simulink model "PID_LOOP_2024a"  (R2024a)
settings: Solver=FixedStepAuto  StartTime=0.0  StopTime=100  FixedStep=dt  RelTol=1e-3
model workspace (MAT data in the model file):
  Drag_Constants = 1
  mass = [5.51 5.51 5.51 1 1 1]
  mass_6a = [5 5 5 1 1 1]
values from neighbouring files (symbols this model uses):
  drag_wrench = [ ... (first row only)    [constants.m]    (also in constants.mat = [0.41 0 0 0 0 0 0 0.5 0 0 0 0 ... (36 elements, 6x6)])
  g = 9.8067    [constants.m]    (also in constants.mat = 9.80665)
  m = mc + mp    (= 6)    [calculate_inertia.m]    (also in constants.mat = 5.51; mass_properties.mat = 10)
  states_desired = [x_des;E_des]    [init.m]
  volume = 0.0074    [constants.m]    (also in constants.mat = 0.0073741788)
  volume_center = [0, 0, -0.07]    [constants.m]    (also in constants.mat = [0 0 0.1])
  water_density = 997    [constants.m]    (also in constants.mat = 1000)
  wrench = eval(w)    [calculate_wrench.m]    (also in constants.m = geometry_properties.wrench; constants.mat = [0 0 0 0 -0.7071 -0.7071 -0.7071 -0.7071 0 0 0 0 ... (48 ele; geometry_properties.mat = [0 0 -1 0.22 0.25 0 0 0 -1 -0.22 0.25 0 ... (48 elements, 6x; wrench.m)
undefined symbols (not defined in the file or in its folder): E0_est, kd, ki, kp, P, pwm_stop, v0_e_est, x0_e_est
libraries: slpidlib x7, simulink x3, shared6dof x1, sharedTrackingLibrary x1
settings Model: Creator=zenyn  LastModifiedBy=kjhaydon
settings DataIOCC: LoggingToFile=on
settings DebuggingCC: UnderSpecifiedDimensionMsg=warning

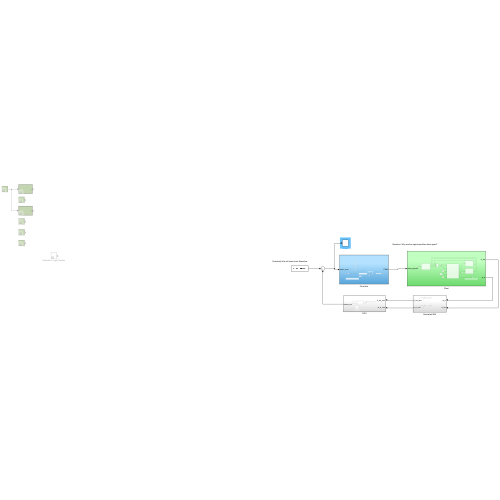
[thumbnail: Simulink's stored preview of the top-level diagram]
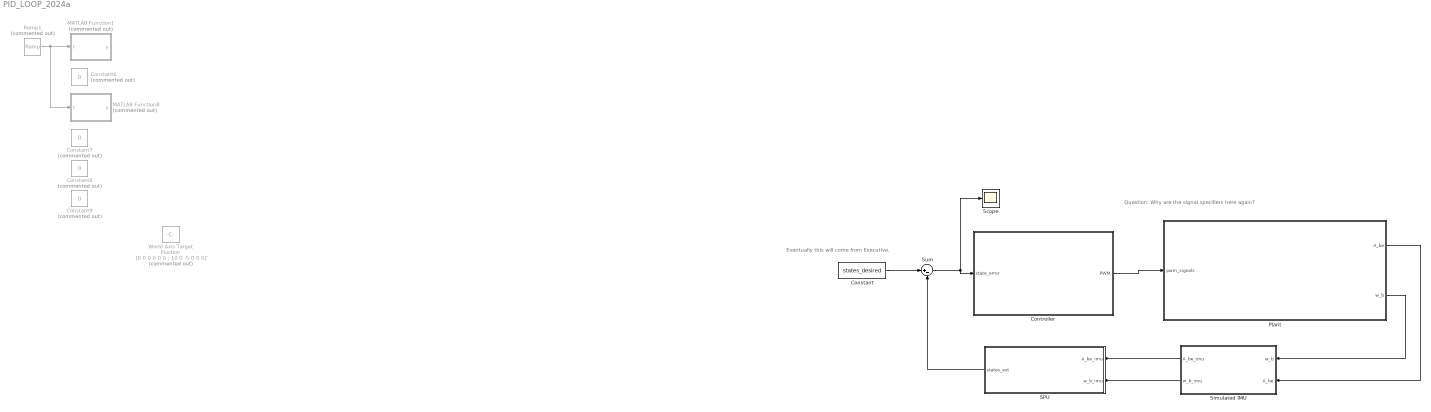
== system PID_LOOP_2024a ==
  note: Eventually this will come from Executive.
  note: Question: Why are the signal specifiers here again?
  Constant : Constant  Value=states_desired
  Constant{6..9} (4 alike) : Constant  Commented=on  Value=0
  Controller : Subsystem
  MATLAB Function1 : MATLAB Function  Commented=on  TreatAsAtomicUnit=on
  MATLAB Function8 : MATLAB Function  Commented=on  TreatAsAtomicUnit=on
  Plant : Subsystem
  Ramp1 : simulink/Sources/Ramp  Commented=on  slope=1  start=0  InitialOutput=0
  SPU : Subsystem
  Scope : Scope
  Simulated IMU : Subsystem
  Sum : Sum  Inputs=|+-
  World Axis Target Position : Constant  Commented=on  Value=[0 0 0 0 0 0 ; 10 0 -5 0 0 0]'
  wires:
  Sum/1 -> Scope/1, Controller/1(state_error)
  Ramp1/1 -> MATLAB Function8/1(t), MATLAB Function1/1(t)
  Simulated IMU/1(A_be_imu) -> SPU/1(A_be_imu)
  SPU/1(states_est) -> Sum/2
  Plant/2(w_b) -> Simulated IMU/1(w_b)
  Plant/1(A_be) -> Simulated IMU/2(A_be)
  Simulated IMU/2(w_b_imu) -> SPU/2(w_b_imu)
  Constant/1 -> Sum/1
  Controller/1(PWM) -> Plant/1(pwm_signals)

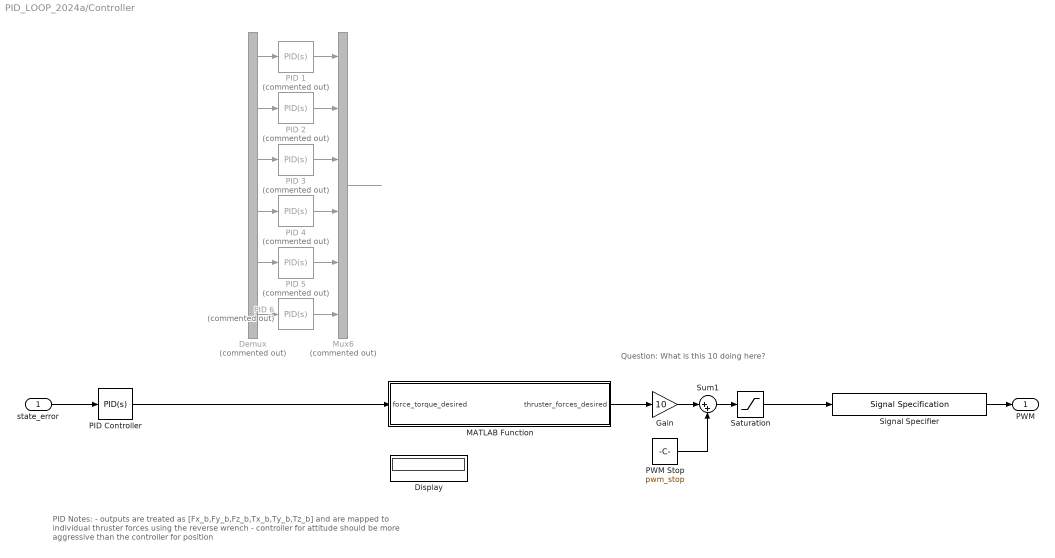
== system PID_LOOP_2024a/Controller ==
  note: Question: What is this 10 doing here?
  note: PID Notes:
      | - outputs are treated as [Fx_b,Fy_b,Fz_b,Tx_b,Ty_b,Tz_b] and are mapped to individual thruster forces using the reverse wrench
      | - controller for attitude should be more aggressive than the controller for position
  state_error : Inport
  Demux : Demux  Commented=on  Outputs=6
  Display : Display
  Gain : Gain  Gain=10
  MATLAB Function : MATLAB Function  TreatAsAtomicUnit=on
  Mux6 : Mux  Commented=on  Inputs=6
  PID 1 : slpidlib/PID Controller  Commented=on  Controller=PID  Form=Parallel  TimeDomain=Continuous-time  UseExternalTs=off  SampleTime=-1  IntegratorMethod=Forward Euler  FilterMethod=Forward Euler  ControllerParametersSource=internal  P=50  I=1  UseKiTs=off  D=80  UseExternalDerivativeSource=off  N=100  UseFilter=on  TunerSelectOption=Transfer Function Based (PID Tuner App)  InitialConditionSource=internal  InitialConditionForIntegrator=0  InitialConditionForFilter=0  DifferentiatorICPrevScaledInput=0  ExternalReset=none  TrackingMode=off  Kt=1  LimitOutput=off  SatLimitsSource=internal  UpperSaturationLimit=inf  LowerSaturationLimit=-inf  LinearizeAsGain=on  AntiWindupMode=none  Kb=1  LimitIntegrator=off  UpperIntegratorSaturationLimit=inf  LowerIntegratorSaturationLimit=-inf  POutMin=[]  POutMax=[]  IOutMin=[]  IOutMax=[]  DOutMin=[]  DOutMax=[]  NOutMin=[]  NOutMax=[]  SumOutMin=[]  SumOutMax=[]  SaturationOutMin=[]  SaturationOutMax=[]  PParamMin=[]  PParamMax=[]  IParamMin=[]  IParamMax=[]  DParamMin=[]  DParamMax=[]  NParamMin=[]  NParamMax=[]  KbParamMin=[]  KbParamMax=[]  KtParamMin=[]  KtParamMax=[]  KbOutMin=[]  KbOutMax=[]  KtOutMin=[]  KtOutMax=[]  IntegratorOutMin=[]  IntegratorOutMax=[]  FilterOutMin=[]  FilterOutMax=[]  SumI1OutMin=[]  SumI1OutMax=[]  SumI2OutMin=[]  SumI2OutMax=[]  SumI3OutMin=[]  SumI3OutMax=[]  SumI4OutMin=[]  SumI4OutMax=[]  SumDOutMin=[]  SumDOutMax=[]  DifferentiatorOutMin=[]  DifferentiatorOutMax=[]  FilterDiffOutCoefMin=[]  FilterDiffOutCoefMax=[]  ReciprocalOutMin=[]  ReciprocalOutMax=[]  SumDenOutMin=[]  SumDenOutMax=[]  SumNumOutMin=[]  SumNumOutMax=[]  DivideOutMin=[]  DivideOutMax=[]  UdiffTsProdOutMin=[]  UdiffTsProdOutMax=[]  NTsProdOutMin=[]  NTsProdOutMax=[]  UintegralTsProdOutMin=[]  UintegralTsProdOutMax=[]  UngainTsProdOutMin=[]  UngainTsProdOutMax=[]  ClampingZeroOutDataTypeStr=Inherit: Inherit via back propagation  ClampingZeroOutMin=[]  ClampingZeroOutMax=[]  FilterDenConstantOutDataTypeStr=Inherit: Inherit via back propagation  FilterDenConstantOutMin=[]  FilterDenConstantOutMax=[]  PCopyOutDataTypeStr=Inherit: Inherit via back propagation  PCopyOutMin=[]  PCopyOutMax=[]  NCopyOutDataTypeStr=Inherit: Inherit via back propagation  NCopyOutMin=[]  NCopyOutMax=[]  IntegratorContinuousStateAttributes=''  IntegratorStateMustResolveToSignalObject=off  IntegratorRTWStateStorageClass=Auto  FilterContinuousStateAttributes=''  FilterStateMustResolveToSignalObject=off  FilterRTWStateStorageClass=Auto  ParallelPVariant=InternalParameters  IdealPVariant=Disabled  IVariant=InternalParameters  DVariant=InternalParameters  IntegratorVariant=Continuous  SatVariant=Disabled  AWVariant=Passthrough  PCopyVariant=Disabled  TRVariant=Disabled  FdbkBlocksVariant=Forward  IdealPFdbkVariant=Disabled  SatFdbkVariant=Disabled  DerivativeFilterVariant=ContFilter  NVariant=InternalParameters  NCopyVariant=Disabled  FilterICVariant=InternalICsFilter  IntegratorICVariant=InternalICs  ExternalResetVariant=Disabled  TRSumVariant=Passthrough  SumFdbkVariant=Disabled  SumVariant=Sum_PID  TsampFilterVariant=InternalTs  TsampNgainVariant=Passthrough  TsampIntegralVariant=Disabled_SignalSpec  ExternalSaturationOutDataTypeStr=Inherit: Same as second input  DerivativeSourceVariant=ErrorSignal
  PID 2 : slpidlib/PID Controller  Commented=on  Controller=PID  Form=Parallel  TimeDomain=Continuous-time  UseExternalTs=off  SampleTime=-1  IntegratorMethod=Forward Euler  FilterMethod=Forward Euler  ControllerParametersSource=internal  P=20  I=1  UseKiTs=off  D=20  UseExternalDerivativeSource=off  N=100  UseFilter=on  TunerSelectOption=Transfer Function Based (PID Tuner App)  InitialConditionSource=internal  InitialConditionForIntegrator=0  InitialConditionForFilter=0  DifferentiatorICPrevScaledInput=0  ExternalReset=none  TrackingMode=off  Kt=1  LimitOutput=off  SatLimitsSource=internal  UpperSaturationLimit=inf  LowerSaturationLimit=-inf  LinearizeAsGain=on  AntiWindupMode=none  Kb=1  LimitIntegrator=off  UpperIntegratorSaturationLimit=inf  LowerIntegratorSaturationLimit=-inf  POutMin=[]  POutMax=[]  IOutMin=[]  IOutMax=[]  DOutMin=[]  DOutMax=[]  NOutMin=[]  NOutMax=[]  SumOutMin=[]  SumOutMax=[]  SaturationOutMin=[]  SaturationOutMax=[]  PParamMin=[]  PParamMax=[]  IParamMin=[]  IParamMax=[]  DParamMin=[]  DParamMax=[]  NParamMin=[]  NParamMax=[]  KbParamMin=[]  KbParamMax=[]  KtParamMin=[]  KtParamMax=[]  KbOutMin=[]  KbOutMax=[]  KtOutMin=[]  KtOutMax=[]  IntegratorOutMin=[]  IntegratorOutMax=[]  FilterOutMin=[]  FilterOutMax=[]  SumI1OutMin=[]  SumI1OutMax=[]  SumI2OutMin=[]  SumI2OutMax=[]  SumI3OutMin=[]  SumI3OutMax=[]  SumI4OutMin=[]  SumI4OutMax=[]  SumDOutMin=[]  SumDOutMax=[]  DifferentiatorOutMin=[]  DifferentiatorOutMax=[]  FilterDiffOutCoefMin=[]  FilterDiffOutCoefMax=[]  ReciprocalOutMin=[]  ReciprocalOutMax=[]  SumDenOutMin=[]  SumDenOutMax=[]  SumNumOutMin=[]  SumNumOutMax=[]  DivideOutMin=[]  DivideOutMax=[]  UdiffTsProdOutMin=[]  UdiffTsProdOutMax=[]  NTsProdOutMin=[]  NTsProdOutMax=[]  UintegralTsProdOutMin=[]  UintegralTsProdOutMax=[]  UngainTsProdOutMin=[]  UngainTsProdOutMax=[]  ClampingZeroOutDataTypeStr=Inherit: Inherit via back propagation  ClampingZeroOutMin=[]  ClampingZeroOutMax=[]  FilterDenConstantOutDataTypeStr=Inherit: Inherit via back propagation  FilterDenConstantOutMin=[]  FilterDenConstantOutMax=[]  PCopyOutDataTypeStr=Inherit: Inherit via back propagation  PCopyOutMin=[]  PCopyOutMax=[]  NCopyOutDataTypeStr=Inherit: Inherit via back propagation  NCopyOutMin=[]  NCopyOutMax=[]  IntegratorContinuousStateAttributes=''  IntegratorStateMustResolveToSignalObject=off  IntegratorRTWStateStorageClass=Auto  FilterContinuousStateAttributes=''  FilterStateMustResolveToSignalObject=off  FilterRTWStateStorageClass=Auto  ParallelPVariant=InternalParameters  IdealPVariant=Disabled  IVariant=InternalParameters  DVariant=InternalParameters  IntegratorVariant=Continuous  SatVariant=Disabled  AWVariant=Passthrough  PCopyVariant=Disabled  TRVariant=Disabled  FdbkBlocksVariant=Forward  IdealPFdbkVariant=Disabled  SatFdbkVariant=Disabled  DerivativeFilterVariant=ContFilter  NVariant=InternalParameters  NCopyVariant=Disabled  FilterICVariant=InternalICsFilter  IntegratorICVariant=InternalICs  ExternalResetVariant=Disabled  TRSumVariant=Passthrough  SumFdbkVariant=Disabled  SumVariant=Sum_PID  TsampFilterVariant=InternalTs  TsampNgainVariant=Passthrough  TsampIntegralVariant=Disabled_SignalSpec  ExternalSaturationOutDataTypeStr=Inherit: Same as second input  DerivativeSourceVariant=ErrorSignal
  PID 3 : slpidlib/PID Controller  Commented=on  Controller=PID  Form=Parallel  TimeDomain=Continuous-time  UseExternalTs=off  SampleTime=-1  IntegratorMethod=Forward Euler  FilterMethod=Forward Euler  ControllerParametersSource=internal  P=40  I=1  UseKiTs=off  D=40  UseExternalDerivativeSource=off  N=100  UseFilter=on  TunerSelectOption=Transfer Function Based (PID Tuner App)  InitialConditionSource=internal  InitialConditionForIntegrator=0  InitialConditionForFilter=0  DifferentiatorICPrevScaledInput=0  ExternalReset=none  TrackingMode=off  Kt=1  LimitOutput=off  SatLimitsSource=internal  UpperSaturationLimit=inf  LowerSaturationLimit=-inf  LinearizeAsGain=on  AntiWindupMode=none  Kb=1  LimitIntegrator=off  UpperIntegratorSaturationLimit=inf  LowerIntegratorSaturationLimit=-inf  POutMin=[]  POutMax=[]  IOutMin=[]  IOutMax=[]  DOutMin=[]  DOutMax=[]  NOutMin=[]  NOutMax=[]  SumOutMin=[]  SumOutMax=[]  SaturationOutMin=[]  SaturationOutMax=[]  PParamMin=[]  PParamMax=[]  IParamMin=[]  IParamMax=[]  DParamMin=[]  DParamMax=[]  NParamMin=[]  NParamMax=[]  KbParamMin=[]  KbParamMax=[]  KtParamMin=[]  KtParamMax=[]  KbOutMin=[]  KbOutMax=[]  KtOutMin=[]  KtOutMax=[]  IntegratorOutMin=[]  IntegratorOutMax=[]  FilterOutMin=[]  FilterOutMax=[]  SumI1OutMin=[]  SumI1OutMax=[]  SumI2OutMin=[]  SumI2OutMax=[]  SumI3OutMin=[]  SumI3OutMax=[]  SumI4OutMin=[]  SumI4OutMax=[]  SumDOutMin=[]  SumDOutMax=[]  DifferentiatorOutMin=[]  DifferentiatorOutMax=[]  FilterDiffOutCoefMin=[]  FilterDiffOutCoefMax=[]  ReciprocalOutMin=[]  ReciprocalOutMax=[]  SumDenOutMin=[]  SumDenOutMax=[]  SumNumOutMin=[]  SumNumOutMax=[]  DivideOutMin=[]  DivideOutMax=[]  UdiffTsProdOutMin=[]  UdiffTsProdOutMax=[]  NTsProdOutMin=[]  NTsProdOutMax=[]  UintegralTsProdOutMin=[]  UintegralTsProdOutMax=[]  UngainTsProdOutMin=[]  UngainTsProdOutMax=[]  ClampingZeroOutDataTypeStr=Inherit: Inherit via back propagation  ClampingZeroOutMin=[]  ClampingZeroOutMax=[]  FilterDenConstantOutDataTypeStr=Inherit: Inherit via back propagation  FilterDenConstantOutMin=[]  FilterDenConstantOutMax=[]  PCopyOutDataTypeStr=Inherit: Inherit via back propagation  PCopyOutMin=[]  PCopyOutMax=[]  NCopyOutDataTypeStr=Inherit: Inherit via back propagation  NCopyOutMin=[]  NCopyOutMax=[]  IntegratorContinuousStateAttributes=''  IntegratorStateMustResolveToSignalObject=off  IntegratorRTWStateStorageClass=Auto  FilterContinuousStateAttributes=''  FilterStateMustResolveToSignalObject=off  FilterRTWStateStorageClass=Auto  ParallelPVariant=InternalParameters  IdealPVariant=Disabled  IVariant=InternalParameters  DVariant=InternalParameters  IntegratorVariant=Continuous  SatVariant=Disabled  AWVariant=Passthrough  PCopyVariant=Disabled  TRVariant=Disabled  FdbkBlocksVariant=Forward  IdealPFdbkVariant=Disabled  SatFdbkVariant=Disabled  DerivativeFilterVariant=ContFilter  NVariant=InternalParameters  NCopyVariant=Disabled  FilterICVariant=InternalICsFilter  IntegratorICVariant=InternalICs  ExternalResetVariant=Disabled  TRSumVariant=Passthrough  SumFdbkVariant=Disabled  SumVariant=Sum_PID  TsampFilterVariant=InternalTs  TsampNgainVariant=Passthrough  TsampIntegralVariant=Disabled_SignalSpec  ExternalSaturationOutDataTypeStr=Inherit: Same as second input  DerivativeSourceVariant=ErrorSignal
  PID 4 : slpidlib/PID Controller  Commented=on  Controller=PID  Form=Parallel  TimeDomain=Continuous-time  UseExternalTs=off  SampleTime=-1  IntegratorMethod=Forward Euler  FilterMethod=Forward Euler  ControllerParametersSource=internal  P=20  I=1  UseKiTs=off  D=20  UseExternalDerivativeSource=off  N=100  UseFilter=on  TunerSelectOption=Transfer Function Based (PID Tuner App)  InitialConditionSource=internal  InitialConditionForIntegrator=0  InitialConditionForFilter=0  DifferentiatorICPrevScaledInput=0  ExternalReset=none  TrackingMode=off  Kt=1  LimitOutput=off  SatLimitsSource=internal  UpperSaturationLimit=inf  LowerSaturationLimit=-inf  LinearizeAsGain=on  AntiWindupMode=none  Kb=1  LimitIntegrator=off  UpperIntegratorSaturationLimit=inf  LowerIntegratorSaturationLimit=-inf  POutMin=[]  POutMax=[]  IOutMin=[]  IOutMax=[]  DOutMin=[]  DOutMax=[]  NOutMin=[]  NOutMax=[]  SumOutMin=[]  SumOutMax=[]  SaturationOutMin=[]  SaturationOutMax=[]  PParamMin=[]  PParamMax=[]  IParamMin=[]  IParamMax=[]  DParamMin=[]  DParamMax=[]  NParamMin=[]  NParamMax=[]  KbParamMin=[]  KbParamMax=[]  KtParamMin=[]  KtParamMax=[]  KbOutMin=[]  KbOutMax=[]  KtOutMin=[]  KtOutMax=[]  IntegratorOutMin=[]  IntegratorOutMax=[]  FilterOutMin=[]  FilterOutMax=[]  SumI1OutMin=[]  SumI1OutMax=[]  SumI2OutMin=[]  SumI2OutMax=[]  SumI3OutMin=[]  SumI3OutMax=[]  SumI4OutMin=[]  SumI4OutMax=[]  SumDOutMin=[]  SumDOutMax=[]  DifferentiatorOutMin=[]  DifferentiatorOutMax=[]  FilterDiffOutCoefMin=[]  FilterDiffOutCoefMax=[]  ReciprocalOutMin=[]  ReciprocalOutMax=[]  SumDenOutMin=[]  SumDenOutMax=[]  SumNumOutMin=[]  SumNumOutMax=[]  DivideOutMin=[]  DivideOutMax=[]  UdiffTsProdOutMin=[]  UdiffTsProdOutMax=[]  NTsProdOutMin=[]  NTsProdOutMax=[]  UintegralTsProdOutMin=[]  UintegralTsProdOutMax=[]  UngainTsProdOutMin=[]  UngainTsProdOutMax=[]  ClampingZeroOutDataTypeStr=Inherit: Inherit via back propagation  ClampingZeroOutMin=[]  ClampingZeroOutMax=[]  FilterDenConstantOutDataTypeStr=Inherit: Inherit via back propagation  FilterDenConstantOutMin=[]  FilterDenConstantOutMax=[]  PCopyOutDataTypeStr=Inherit: Inherit via back propagation  PCopyOutMin=[]  PCopyOutMax=[]  NCopyOutDataTypeStr=Inherit: Inherit via back propagation  NCopyOutMin=[]  NCopyOutMax=[]  IntegratorContinuousStateAttributes=''  IntegratorStateMustResolveToSignalObject=off  IntegratorRTWStateStorageClass=Auto  FilterContinuousStateAttributes=''  FilterStateMustResolveToSignalObject=off  FilterRTWStateStorageClass=Auto  ParallelPVariant=InternalParameters  IdealPVariant=Disabled  IVariant=InternalParameters  DVariant=InternalParameters  IntegratorVariant=Continuous  SatVariant=Disabled  AWVariant=Passthrough  PCopyVariant=Disabled  TRVariant=Disabled  FdbkBlocksVariant=Forward  IdealPFdbkVariant=Disabled  SatFdbkVariant=Disabled  DerivativeFilterVariant=ContFilter  NVariant=InternalParameters  NCopyVariant=Disabled  FilterICVariant=InternalICsFilter  IntegratorICVariant=InternalICs  ExternalResetVariant=Disabled  TRSumVariant=Passthrough  SumFdbkVariant=Disabled  SumVariant=Sum_PID  TsampFilterVariant=InternalTs  TsampNgainVariant=Passthrough  TsampIntegralVariant=Disabled_SignalSpec  ExternalSaturationOutDataTypeStr=Inherit: Same as second input  DerivativeSourceVariant=ErrorSignal
  PID 5 : slpidlib/PID Controller  Commented=on  Controller=PID  Form=Parallel  TimeDomain=Continuous-time  UseExternalTs=off  SampleTime=-1  IntegratorMethod=Forward Euler  FilterMethod=Forward Euler  ControllerParametersSource=internal  P=20  I=1  UseKiTs=off  D=50  UseExternalDerivativeSource=off  N=100  UseFilter=on  TunerSelectOption=Transfer Function Based (PID Tuner App)  InitialConditionSource=internal  InitialConditionForIntegrator=0  InitialConditionForFilter=0  DifferentiatorICPrevScaledInput=0  ExternalReset=none  TrackingMode=off  Kt=1  LimitOutput=off  SatLimitsSource=internal  UpperSaturationLimit=inf  LowerSaturationLimit=-inf  LinearizeAsGain=on  AntiWindupMode=none  Kb=1  LimitIntegrator=off  UpperIntegratorSaturationLimit=inf  LowerIntegratorSaturationLimit=-inf  POutMin=[]  POutMax=[]  IOutMin=[]  IOutMax=[]  DOutMin=[]  DOutMax=[]  NOutMin=[]  NOutMax=[]  SumOutMin=[]  SumOutMax=[]  SaturationOutMin=[]  SaturationOutMax=[]  PParamMin=[]  PParamMax=[]  IParamMin=[]  IParamMax=[]  DParamMin=[]  DParamMax=[]  NParamMin=[]  NParamMax=[]  KbParamMin=[]  KbParamMax=[]  KtParamMin=[]  KtParamMax=[]  KbOutMin=[]  KbOutMax=[]  KtOutMin=[]  KtOutMax=[]  IntegratorOutMin=[]  IntegratorOutMax=[]  FilterOutMin=[]  FilterOutMax=[]  SumI1OutMin=[]  SumI1OutMax=[]  SumI2OutMin=[]  SumI2OutMax=[]  SumI3OutMin=[]  SumI3OutMax=[]  SumI4OutMin=[]  SumI4OutMax=[]  SumDOutMin=[]  SumDOutMax=[]  DifferentiatorOutMin=[]  DifferentiatorOutMax=[]  FilterDiffOutCoefMin=[]  FilterDiffOutCoefMax=[]  ReciprocalOutMin=[]  ReciprocalOutMax=[]  SumDenOutMin=[]  SumDenOutMax=[]  SumNumOutMin=[]  SumNumOutMax=[]  DivideOutMin=[]  DivideOutMax=[]  UdiffTsProdOutMin=[]  UdiffTsProdOutMax=[]  NTsProdOutMin=[]  NTsProdOutMax=[]  UintegralTsProdOutMin=[]  UintegralTsProdOutMax=[]  UngainTsProdOutMin=[]  UngainTsProdOutMax=[]  ClampingZeroOutDataTypeStr=Inherit: Inherit via back propagation  ClampingZeroOutMin=[]  ClampingZeroOutMax=[]  FilterDenConstantOutDataTypeStr=Inherit: Inherit via back propagation  FilterDenConstantOutMin=[]  FilterDenConstantOutMax=[]  PCopyOutDataTypeStr=Inherit: Inherit via back propagation  PCopyOutMin=[]  PCopyOutMax=[]  NCopyOutDataTypeStr=Inherit: Inherit via back propagation  NCopyOutMin=[]  NCopyOutMax=[]  IntegratorContinuousStateAttributes=''  IntegratorStateMustResolveToSignalObject=off  IntegratorRTWStateStorageClass=Auto  FilterContinuousStateAttributes=''  FilterStateMustResolveToSignalObject=off  FilterRTWStateStorageClass=Auto  ParallelPVariant=InternalParameters  IdealPVariant=Disabled  IVariant=InternalParameters  DVariant=InternalParameters  IntegratorVariant=Continuous  SatVariant=Disabled  AWVariant=Passthrough  PCopyVariant=Disabled  TRVariant=Disabled  FdbkBlocksVariant=Forward  IdealPFdbkVariant=Disabled  SatFdbkVariant=Disabled  DerivativeFilterVariant=ContFilter  NVariant=InternalParameters  NCopyVariant=Disabled  FilterICVariant=InternalICsFilter  IntegratorICVariant=InternalICs  ExternalResetVariant=Disabled  TRSumVariant=Passthrough  SumFdbkVariant=Disabled  SumVariant=Sum_PID  TsampFilterVariant=InternalTs  TsampNgainVariant=Passthrough  TsampIntegralVariant=Disabled_SignalSpec  ExternalSaturationOutDataTypeStr=Inherit: Same as second input  DerivativeSourceVariant=ErrorSignal
  PID 6 : slpidlib/PID Controller  Commented=on  Controller=PID  Form=Parallel  TimeDomain=Continuous-time  UseExternalTs=off  SampleTime=-1  IntegratorMethod=Forward Euler  FilterMethod=Forward Euler  ControllerParametersSource=internal  P=5  I=1  UseKiTs=off  D=5  UseExternalDerivativeSource=off  N=100  UseFilter=on  TunerSelectOption=Transfer Function Based (PID Tuner App)  InitialConditionSource=internal  InitialConditionForIntegrator=0  InitialConditionForFilter=0  DifferentiatorICPrevScaledInput=0  ExternalReset=none  TrackingMode=off  Kt=1  LimitOutput=off  SatLimitsSource=internal  UpperSaturationLimit=inf  LowerSaturationLimit=-inf  LinearizeAsGain=on  AntiWindupMode=none  Kb=1  LimitIntegrator=off  UpperIntegratorSaturationLimit=inf  LowerIntegratorSaturationLimit=-inf  POutMin=[]  POutMax=[]  IOutMin=[]  IOutMax=[]  DOutMin=[]  DOutMax=[]  NOutMin=[]  NOutMax=[]  SumOutMin=[]  SumOutMax=[]  SaturationOutMin=[]  SaturationOutMax=[]  PParamMin=[]  PParamMax=[]  IParamMin=[]  IParamMax=[]  DParamMin=[]  DParamMax=[]  NParamMin=[]  NParamMax=[]  KbParamMin=[]  KbParamMax=[]  KtParamMin=[]  KtParamMax=[]  KbOutMin=[]  KbOutMax=[]  KtOutMin=[]  KtOutMax=[]  IntegratorOutMin=[]  IntegratorOutMax=[]  FilterOutMin=[]  FilterOutMax=[]  SumI1OutMin=[]  SumI1OutMax=[]  SumI2OutMin=[]  SumI2OutMax=[]  SumI3OutMin=[]  SumI3OutMax=[]  SumI4OutMin=[]  SumI4OutMax=[]  SumDOutMin=[]  SumDOutMax=[]  DifferentiatorOutMin=[]  DifferentiatorOutMax=[]  FilterDiffOutCoefMin=[]  FilterDiffOutCoefMax=[]  ReciprocalOutMin=[]  ReciprocalOutMax=[]  SumDenOutMin=[]  SumDenOutMax=[]  SumNumOutMin=[]  SumNumOutMax=[]  DivideOutMin=[]  DivideOutMax=[]  UdiffTsProdOutMin=[]  UdiffTsProdOutMax=[]  NTsProdOutMin=[]  NTsProdOutMax=[]  UintegralTsProdOutMin=[]  UintegralTsProdOutMax=[]  UngainTsProdOutMin=[]  UngainTsProdOutMax=[]  ClampingZeroOutDataTypeStr=Inherit: Inherit via back propagation  ClampingZeroOutMin=[]  ClampingZeroOutMax=[]  FilterDenConstantOutDataTypeStr=Inherit: Inherit via back propagation  FilterDenConstantOutMin=[]  FilterDenConstantOutMax=[]  PCopyOutDataTypeStr=Inherit: Inherit via back propagation  PCopyOutMin=[]  PCopyOutMax=[]  NCopyOutDataTypeStr=Inherit: Inherit via back propagation  NCopyOutMin=[]  NCopyOutMax=[]  IntegratorContinuousStateAttributes=''  IntegratorStateMustResolveToSignalObject=off  IntegratorRTWStateStorageClass=Auto  FilterContinuousStateAttributes=''  FilterStateMustResolveToSignalObject=off  FilterRTWStateStorageClass=Auto  ParallelPVariant=InternalParameters  IdealPVariant=Disabled  IVariant=InternalParameters  DVariant=InternalParameters  IntegratorVariant=Continuous  SatVariant=Disabled  AWVariant=Passthrough  PCopyVariant=Disabled  TRVariant=Disabled  FdbkBlocksVariant=Forward  IdealPFdbkVariant=Disabled  SatFdbkVariant=Disabled  DerivativeFilterVariant=ContFilter  NVariant=InternalParameters  NCopyVariant=Disabled  FilterICVariant=InternalICsFilter  IntegratorICVariant=InternalICs  ExternalResetVariant=Disabled  TRSumVariant=Passthrough  SumFdbkVariant=Disabled  SumVariant=Sum_PID  TsampFilterVariant=InternalTs  TsampNgainVariant=Passthrough  TsampIntegralVariant=Disabled_SignalSpec  ExternalSaturationOutDataTypeStr=Inherit: Same as second input  DerivativeSourceVariant=ErrorSignal
  PID Controller : slpidlib/PID Controller  Controller=PID  Form=Parallel  TimeDomain=Continuous-time  UseExternalTs=off  SampleTime=-1  IntegratorMethod=Forward Euler  FilterMethod=Forward Euler  ControllerParametersSource=internal  P=kp  I=ki  UseKiTs=off  D=kd  UseExternalDerivativeSource=off  N=100  UseFilter=on  TunerSelectOption=Frequency Response Based  InitialConditionSource=internal  InitialConditionForIntegrator=0  InitialConditionForFilter=0  DifferentiatorICPrevScaledInput=0  ExternalReset=none  TrackingMode=off  Kt=1  LimitOutput=off  SatLimitsSource=internal  UpperSaturationLimit=inf  LowerSaturationLimit=-inf  LinearizeAsGain=on  AntiWindupMode=none  Kb=1  LimitIntegrator=off  UpperIntegratorSaturationLimit=inf  LowerIntegratorSaturationLimit=-inf  POutMin=[]  POutMax=[]  IOutMin=[]  IOutMax=[]  DOutMin=[]  DOutMax=[]  NOutMin=[]  NOutMax=[]  SumOutMin=[]  SumOutMax=[]  SaturationOutMin=[]  SaturationOutMax=[]  PParamMin=[]  PParamMax=[]  IParamMin=[]  IParamMax=[]  DParamMin=[]  DParamMax=[]  NParamMin=[]  NParamMax=[]  KbParamMin=[]  KbParamMax=[]  KtParamMin=[]  KtParamMax=[]  KbOutMin=[]  KbOutMax=[]  KtOutMin=[]  KtOutMax=[]  IntegratorOutMin=[]  IntegratorOutMax=[]  FilterOutMin=[]  FilterOutMax=[]  SumI1OutMin=[]  SumI1OutMax=[]  SumI2OutMin=[]  SumI2OutMax=[]  SumI3OutMin=[]  SumI3OutMax=[]  SumI4OutMin=[]  SumI4OutMax=[]  SumDOutMin=[]  SumDOutMax=[]  DifferentiatorOutMin=[]  DifferentiatorOutMax=[]  FilterDiffOutCoefMin=[]  FilterDiffOutCoefMax=[]  ReciprocalOutMin=[]  ReciprocalOutMax=[]  SumDenOutMin=[]  SumDenOutMax=[]  SumNumOutMin=[]  SumNumOutMax=[]  DivideOutMin=[]  DivideOutMax=[]  UdiffTsProdOutMin=[]  UdiffTsProdOutMax=[]  NTsProdOutMin=[]  NTsProdOutMax=[]  UintegralTsProdOutMin=[]  UintegralTsProdOutMax=[]  UngainTsProdOutMin=[]  UngainTsProdOutMax=[]  ClampingZeroOutDataTypeStr=Inherit: Inherit via back propagation  ClampingZeroOutMin=[]  ClampingZeroOutMax=[]  FilterDenConstantOutDataTypeStr=Inherit: Inherit via back propagation  FilterDenConstantOutMin=[]  FilterDenConstantOutMax=[]  PCopyOutDataTypeStr=Inherit: Inherit via back propagation  PCopyOutMin=[]  PCopyOutMax=[]  NCopyOutDataTypeStr=Inherit: Inherit via back propagation  NCopyOutMin=[]  NCopyOutMax=[]  IntegratorContinuousStateAttributes=''  IntegratorStateMustResolveToSignalObject=off  IntegratorRTWStateStorageClass=Auto  FilterContinuousStateAttributes=''  FilterStateMustResolveToSignalObject=off  FilterRTWStateStorageClass=Auto  ParallelPVariant=InternalParameters  IdealPVariant=Disabled  IVariant=InternalParameters  DVariant=InternalParameters  IntegratorVariant=Continuous  SatVariant=Disabled  AWVariant=Passthrough  PCopyVariant=Disabled  TRVariant=Disabled  FdbkBlocksVariant=Forward  IdealPFdbkVariant=Disabled  SatFdbkVariant=Disabled  DerivativeFilterVariant=ContFilter  NVariant=InternalParameters  NCopyVariant=Disabled  FilterICVariant=InternalICsFilter  IntegratorICVariant=InternalICs  ExternalResetVariant=Disabled  TRSumVariant=Passthrough  SumFdbkVariant=Disabled  SumVariant=Sum_PID  TsampFilterVariant=InternalTs  TsampNgainVariant=Passthrough  TsampIntegralVariant=Disabled_SignalSpec  ExternalSaturationOutDataTypeStr=Inherit: Same as second input  DerivativeSourceVariant=ErrorSignal
  PWM Stop : Constant  Value=pwm_stop
  Saturation : Saturate  UpperLimit=1900  LowerLimit=1100
  Signal Specifier : SignalSpecification  OutMin=[1200 ]  OutMax=[ 1800 ]  OutDataTypeStr=double  Unit=µs  Dimensions=[8 1]
  Sum1 : Sum  Inputs=|++
  PWM : Outport
  wires:
  Mux6/1 -> ?
  Demux/6 -> PID 6/1
  Demux/5 -> PID 5/1
  Demux/4 -> PID 4/1
  Demux/3 -> PID 3/1
  Demux/2 -> PID 2/1
  Demux/1 -> PID 1/1
  PID 1/1 -> Mux6/1
  PID 2/1 -> Mux6/2
  PID 3/1 -> Mux6/3
  PID 4/1 -> Mux6/4
  PID 5/1 -> Mux6/5
  PID 6/1 -> Mux6/6
  PWM Stop/1 -> Sum1/2
  Saturation/1 -> Signal Specifier/1
  Gain/1 -> Sum1/1
  Sum1/1 -> Saturation/1
  MATLAB Function/1(thruster_forces_desired) -> Gain/1
  Signal Specifier/1 -> PWM/1
  state_error/1 -> PID Controller/1
  PID Controller/1 -> MATLAB Function/1(force_torque_desired)

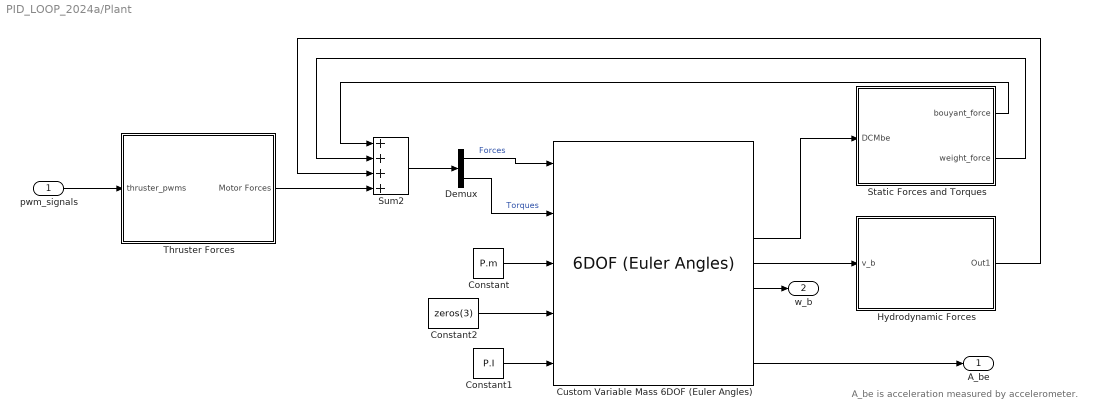
== system PID_LOOP_2024a/Plant ==
  note: A_be is acceleration measured by accelerometer.
  pwm_signals : Inport
  Constant : Constant  Value=P.m
  Constant1 : Constant  Value=P.I
  Constant2 : Constant  Value=zeros(3)
  Custom Variable Mass 6DOF (Euler Angles) : shared6dof/6DOF (Euler Angles)  units=Metric (MKS)  mtype=Custom Variable  rep=Euler Angles  xme_0=x0_e  Vm_0=v0_e  eul_0=E0  pm_0=w0  mass_0=1.0  mass_e=0.5  mass_f=2.0  inertia=eye(3)  inertia_e=eye(3)  inertia_f=2*eye(3)  k_quat=1.0  vre_flag=off  abi_flag=on  aMode=0  xme_statename=''  Vm_statename=''  eul_statename=''  quat_statename=''  pm_statename=''  mass_statename=''
      settings: LibrarySourceBlock=aerolib6dof2/Custom Variable Mass 6DOF (Euler Angles)
  Demux : Demux  Outputs=2
  Hydrodynamic Forces : Subsystem
  Static Forces and Torques : Subsystem
  Sum2 : Sum  Inputs=++++
  Thruster Forces : Subsystem
  A_be : Outport
  w_b : Outport  Port=2
  wires:
  Sum2/1 -> Demux/1
  Demux/1 -> Custom Variable Mass 6DOF (Euler Angles)/1  "Forces"
  Demux/2 -> Custom Variable Mass 6DOF (Euler Angles)/2  "Torques"
  Custom Variable Mass 6DOF (Euler Angles)/9 -> A_be/1
  Constant/1 -> Custom Variable Mass 6DOF (Euler Angles)/3
  Constant1/1 -> Custom Variable Mass 6DOF (Euler Angles)/5
  Constant2/1 -> Custom Variable Mass 6DOF (Euler Angles)/4
  Custom Variable Mass 6DOF (Euler Angles)/5 -> Hydrodynamic Forces/1(v_b)
  Custom Variable Mass 6DOF (Euler Angles)/4 -> Static Forces and Torques/1(DCMbe)
  pwm_signals/1 -> Thruster Forces/1(thruster_pwms)
  Thruster Forces/1(Motor Forces) -> Sum2/4
  Hydrodynamic Forces/1(Out1) -> Sum2/3
  Static Forces and Torques/2(weight_force) -> Sum2/2
  Static Forces and Torques/1(bouyant_force) -> Sum2/1
  Custom Variable Mass 6DOF (Euler Angles)/6 -> w_b/1

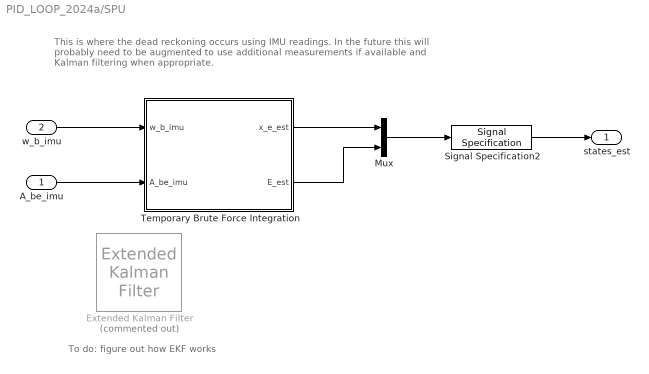
== system PID_LOOP_2024a/SPU ==
  note: To do: figure out how EKF works
  note: This is where the dead reckoning occurs using IMU readings. In the future this will
      | probably need to be augmented to use additional measurements if available and
      | Kalman filtering when appropriate.
  A_be_imu : Inport
  w_b_imu : Inport  Port=2
  Extended Kalman Filter : sharedTrackingLibrary/Extended Kalman Filter  Commented=on  StateTransitionFcn=myStateTransitionFcn  HasStateTransitionJacobianFcn=off  HasAdditiveProcessNoise=Additive  ProcessNoise=1  HasTimeVaryingProcessNoise=off  HasStateTransitionFcnExtraArgument=0  InitialState=0  InitialStateCovariance=1  MeasurementFcn1=myMeasurementFcn  HasMeasurementJacobianFcn1=off  HasMeasurementEnablePort1=off  HasAdditiveMeasurementNoise1=Additive  MeasurementNoise1=1  HasTimeVaryingMeasurementNoise1=off  HasMeasurementFcnExtraArgument1=0  HasMeasurementWrapping1=off  MeasurementFcn2=myMeasurementFcn  HasMeasurementJacobianFcn2=off  HasMeasurementEnablePort2=off  HasAdditiveMeasurementNoise2=Additive  MeasurementNoise2=1  HasTimeVaryingMeasurementNoise2=off  HasMeasurementFcnExtraArgument2=0  HasMeasurementWrapping2=off  MeasurementFcn3=myMeasurementFcn  HasMeasurementJacobianFcn3=off  HasMeasurementEnablePort3=off  HasAdditiveMeasurementNoise3=Additive  MeasurementNoise3=1  HasTimeVaryingMeasurementNoise3=off  HasMeasurementFcnExtraArgument3=0  HasMeasurementWrapping3=off  MeasurementFcn4=myMeasurementFcn  HasMeasurementJacobianFcn4=off  HasMeasurementEnablePort4=off  HasAdditiveMeasurementNoise4=Additive  MeasurementNoise4=1  HasTimeVaryingMeasurementNoise4=off  HasMeasurementFcnExtraArgument4=0  HasMeasurementWrapping4=off  MeasurementFcn5=myMeasurementFcn  HasMeasurementJacobianFcn5=off  HasMeasurementEnablePort5=off  HasAdditiveMeasurementNoise5=Additive  MeasurementNoise5=1  HasTimeVaryingMeasurementNoise5=off  HasMeasurementFcnExtraArgument5=0  HasMeasurementWrapping5=off  EnableMultirate=off  StateTransitionFcnSampleTime=1  MeasurementFcn1SampleTime=1  MeasurementFcn2SampleTime=1  MeasurementFcn3SampleTime=1  MeasurementFcn4SampleTime=1  MeasurementFcn5SampleTime=1  UseCurrentEstimator=on  OutputStateCovariance=off  DataType=double  SampleTime=1  NumberOfMeasurements=1
  Mux : Mux  Inputs=2
  Signal Specification2 : SignalSpecification  Dimensions=[6 1]
  Temporary Brute Force Integration : Subsystem
  states_est : Outport
  wires:
  w_b_imu/1 -> Temporary Brute Force Integration/1(w_b_imu)
  A_be_imu/1 -> Temporary Brute Force Integration/2(A_be_imu)
  Temporary Brute Force Integration/2(E_est) -> Mux/2
  Temporary Brute Force Integration/1(x_e_est) -> Mux/1
  Mux/1 -> Signal Specification2/1
  Signal Specification2/1 -> states_est/1

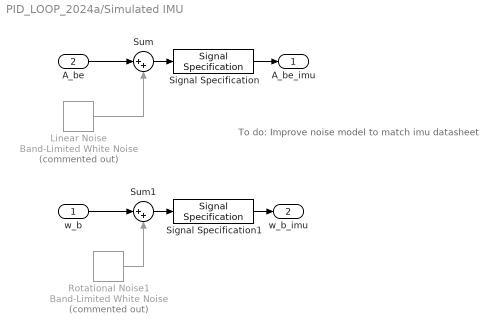
== system PID_LOOP_2024a/Simulated IMU ==
  note: To do: Improve noise model to match imu datasheet
  w_b : Inport
  A_be : Inport  Port=2
  Linear Noise : simulink/Sources/Band-Limited White Noise  Commented=on  Cov=lin_noise  Ts=0.1  seed=[23341]
  Rotational Noise1 : simulink/Sources/Band-Limited White Noise  Commented=on  Cov=rot_noise  Ts=0.1  seed=[23341]
  Signal Specification : SignalSpecification  Dimensions=[3 1]
  Signal Specification1 : SignalSpecification  Dimensions=[3 1]
  Sum : Sum  Inputs=|++
  Sum1 : Sum  Inputs=|++
  A_be_imu : Outport
  w_b_imu : Outport  Port=2
  wires:
  Sum1/1 -> Signal Specification1/1
  Linear Noise/1 -> Sum/2
  Rotational Noise1/1 -> Sum1/2
  A_be/1 -> Sum/1
  w_b/1 -> Sum1/1
  Sum/1 -> Signal Specification/1
  Signal Specification/1 -> A_be_imu/1
  Signal Specification1/1 -> w_b_imu/1

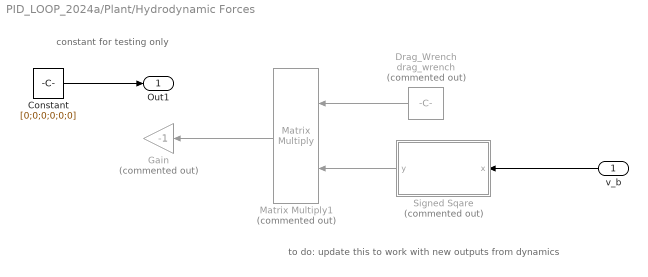
== system PID_LOOP_2024a/Plant/Hydrodynamic Forces ==
  note: to do: update this to work with new outputs from dynamics
  note: constant for testing only
  v_b : Inport
  Constant : Constant  Value=[0;0;0;0;0;0]
  Drag_Wrench : Constant  Commented=on  Value=drag_wrench  VectorParams1D=off
  Gain : Gain  Commented=on  Gain=-1
  Matrix Multiply1 : Product  Commented=on  Multiplication=Matrix(*)
  Signed Sqare : MATLAB Function  Commented=on  TreatAsAtomicUnit=on
  Out1 : Outport
  wires:
  v_b/1 -> Signed Sqare/1(x)
  Matrix Multiply1/1 -> Gain/1
  Constant/1 -> Out1/1
  Drag_Wrench/1 -> Matrix Multiply1/1
  Signed Sqare/1(y) -> Matrix Multiply1/2

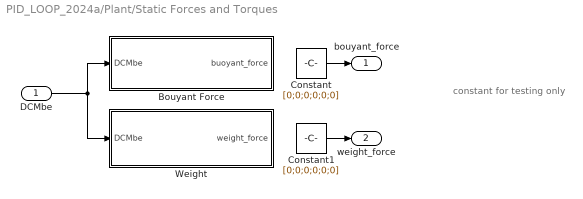
== system PID_LOOP_2024a/Plant/Static Forces and Torques ==
  note: constant for testing only
  DCMbe : Inport
  Bouyant Force : MATLAB Function  TreatAsAtomicUnit=on
  Constant : Constant  Value=[0;0;0;0;0;0]
  Constant1 : Constant  Value=[0;0;0;0;0;0]
  Weight : MATLAB Function  TreatAsAtomicUnit=on
  bouyant_force : Outport
  weight_force : Outport  Port=2
  wires:
  DCMbe/1 -> Weight/1(DCMbe), Bouyant Force/1(DCMbe)
  Constant/1 -> bouyant_force/1
  Constant1/1 -> weight_force/1

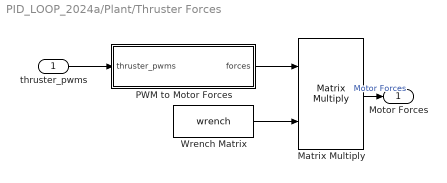
== system PID_LOOP_2024a/Plant/Thruster Forces ==
  thruster_pwms : Inport
  Matrix Multiply : Product  Multiplication=Matrix(*)
  PWM to Motor Forces : MATLAB Function  TreatAsAtomicUnit=on
  Wrench Matrix : Constant  Value=wrench  VectorParams1D=off
  Motor Forces : Outport
  wires:
  Matrix Multiply/1 -> Motor Forces/1  "Motor Forces"
  thruster_pwms/1 -> PWM to Motor Forces/1(thruster_pwms)
  PWM to Motor Forces/1(forces) -> Matrix Multiply/1
  Wrench Matrix/1 -> Matrix Multiply/2

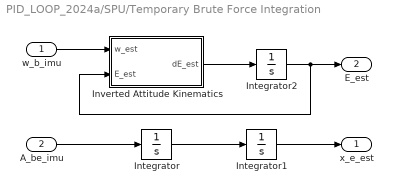
== system PID_LOOP_2024a/SPU/Temporary Brute Force Integration ==
  w_b_imu : Inport
  A_be_imu : Inport  Port=2
  Integrator : Integrator  InitialCondition=v0_e_est
  Integrator1 : Integrator  InitialCondition=x0_e_est
  Integrator2 : Integrator  InitialCondition=E0_est
  Inverted Attitude Kinematics : MATLAB Function  TreatAsAtomicUnit=on
  x_e_est : Outport
  E_est : Outport  Port=2
  wires:
  A_be_imu/1 -> Integrator/1
  Integrator/1 -> Integrator1/1
  w_b_imu/1 -> Inverted Attitude Kinematics/1(w_est)
  Inverted Attitude Kinematics/1(dE_est) -> Integrator2/1
  Integrator2/1 -> E_est/1, Inverted Attitude Kinematics/2(E_est)
  Integrator1/1 -> x_e_est/1

== matlab function PID_LOOP_2024a/Plant/Hydrodynamic Forces/Signed Sqare ==
  data: x input; y output
function y = signed_square(x)
y = x .* abs(x);
end

== matlab function PID_LOOP_2024a/Plant/Thruster Forces/PWM to Motor Forces ==
  data: thruster_pwms input; forces output; P parameter
function forces  = fcn(thruster_pwms,P)
    %{
        This function  uses a polynomial fit to the pwm vs thrust curve 
        for the T200 Thrusters to calculate the 8 thruster force vectors.
    %}
    %preallocate
    forces_kgf = zeros(size(thruster_pwms)); 
    
    
    % First condition: 1100 <= x < 1460
    index_array = (thruster_pwms >= 1100 & thruster_pwms < 1460);

    
    forces_kgf(index_array) = (-1.24422882971549e-8) * thruster_pwms(index_array).^3 ...
                 + (4.02057100632393e-5) * thruster_pwms(index_array).^2 ...
                 - 0.0348619861030835 * thruster_pwms(index_array) ...
                 + 3.90671429105423;
    
    % Second condition: 1460 <= x <= 1540
    index_array = (thruster_pwms >= 1460 & thruster_pwms <= 1540);
    forces_kgf(index_array) = 0;
    
    % Third condition: 1540 < x <= 1900
    index_array = (thruster_pwms > 1540 & thruster_pwms <= 1900);
    forces_kgf(index_array) = (-1.64293565374284e-8) * thruster_pwms(index_array).^3 ...
                 + (9.45962838560648e-5) * thruster_pwms(index_array).^2 ...
                 - 0.170812079190679 * thruster_pwms(index_array) ...
                 + 98.7232373648272;
    
    % Handle out-of-range values
    if any(isnan(forces_kgf))
        error('Some values in x_array are out of the valid range [1100..1900].');
    end

    forces = (forces_kgf/P.g)'; %convert to N
    
end

== matlab function PID_LOOP_2024a/SPU/Temporary Brute Force Integration/Inverted Attitude Kinematics ==
  data: w_est input; dE_est output; E_est input
function dE_est = fcn(w_est,E_est)
%unpack Euler angles
phi = E_est(1);
theta = E_est(2);
psi = E_est(3);

dE_est = [1, sin(phi)*tan(theta), cos(phi)*tan(theta);...
    0, cos(phi), -sin(phi);...
    0, sin(phi)/cos(theta), cos(phi)/cos(theta)]*w_est;

== matlab function PID_LOOP_2024a/Plant/Static Forces and Torques/Bouyant Force ==
  data: DCMbe input; buoyant_force output; g parameter; water_density parameter; volume parameter; volume_center parameter
function buoyant_force = buoyant_force(DCMbe, g, water_density, volume, volume_center)

    % Ensure d is a column vector
    volume_center = volume_center(:);

    % Buoyant force vector in world frame
    b_vector = [0; 0; water_density * -g * volume];

    % Rotate buoyant force to object's frame
    buoyant_force_body = DCMbe * b_vector;

    % Compute torque using cross product τ = d × F_buoyancy
    % (MATLAB cross function works for column vectors)
    torque = cross(-volume_center, buoyant_force_body);

    % Combine force and torque into a single output vector
    buoyant_force = [buoyant_force_body; torque]';
end

== matlab function PID_LOOP_2024a/Plant/Static Forces and Torques/Weight ==
  data: DCMbe input; weight_force output; g parameter; m parameter
function weight_force = weight_force(DCMbe, g, m)

    % Gravity force vector in world frame (downward)
    g_vector = [0; 0; m * g];
    
    % Linear Force
    lin = DCMbe * g_vector;
    % Rotational force
    rot = [0;0;0];
    % Transform gravity force to rotated frame
    weight_force = [lin', rot'];
end

== matlab function PID_LOOP_2024a/Controller/MATLAB Function ==
  data: force_torque_desired input; thruster_forces_desired output; wrench parameter
function thruster_forces_desired = rev_wrench(force_torque_desired, wrench)

inv_wrench = pinv(wrench);
thruster_forces_desired = inv_wrench' * force_torque_desired;

end

== matlab function PID_LOOP_2024a/MATLAB Function1 ==
  data: t input; y output
function y = fcn(t)

if t < 30
    y = t;
elseif t < 60
    y = 30;
else
    y = 90 - t;

end

== matlab function PID_LOOP_2024a/MATLAB Function8 ==
  data: t input; y output
function y = fcn(t)

speed = 30 / 30; 
if t < 30
    y = 0;
elseif t < 60
    y = 30 * speed - t * speed;
else
    y = 30 * speed - 60 * speed;
end
